simulink model "origin_cont"  (R2017b)
settings: Solver=VariableStepAuto  StartTime=0.0  StopTime=3  FixedStep=0.1  RelTol=1e-3
values from neighbouring files (symbols this model uses):
  gama1 = 109    [init.m]    (also in int.m = x(i,1); main.m = 10)
  gama2 = 2.04    [init.m]    (also in int.m = x(i,2); main.m = 10)
  kd = 3000    [PSO_main.m]    (also in init.m = 1000)
  ke = 1000    [PSO_main.m]    (also in init.m = 3000)
libraries: simulink x1
settings Model: Creator=Administrator  LastModifiedBy=Administrator
settings SolverCC: ZeroCrossAlgorithm=Adaptive
settings DebuggingCC: MaxConsecutiveZCsMsg=none
settings RTWCC: GenCodeOnly=on  PackageName=auto_impedance  Toolchain=Microsoft Visual C++ 2017 v15.0 | nmake (64-bit Windows)

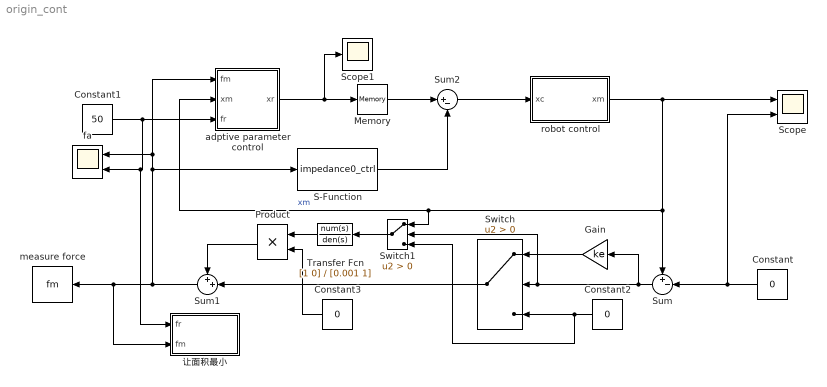
== system origin_cont ==
  Constant : Constant  Value=0
  Constant1 : Constant  Value=50
  Constant2 : Constant  Value=0
  Constant3 : Constant  Value=0
  Gain : Gain  Gain=ke
  Memory : Memory
  Product : Product
  S-Function : S-Function  FunctionName=impedance0_ctrl  Parameters=bd kd  SFunctionDeploymentMode=off  EnableBusSupport=off
  Scope : Scope  NumInputPorts=2
  Scope1 : Scope
  Sum : Sum  Inputs=+-|
  Sum1 : Sum  Inputs=++|
  Sum2 : Sum  Inputs=|+-
  Switch : Switch  Criteria=u2 > Threshold
  Switch1 : Switch  Criteria=u2 > Threshold
  Transfer Fcn : TransferFcn  Numerator=[1 0]  Denominator=[0.001 1]
  adptive parameter control : Subsystem
  fa : Scope  NumInputPorts=2
  "measure force " : ToWorkspace  VariableName=fm  SaveFormat=Timeseries  SampleTime=-1
  robot control : Subsystem
  让面积最小 : Subsystem
  wires:
  robot control/1("xm ") -> Switch1/1, adptive parameter control/2(xm), Sum/1, Scope/1  "xm"
  adptive parameter control/1(xr) -> Memory/1, Scope1/1
  Constant2/1 -> Switch1/3, Switch/3
  Sum2/1 -> robot control/1(xc)
  S-Function/1 -> Sum2/2
  Sum/1 -> Switch1/2, Switch/2, Gain/1
  Gain/1 -> Switch/1
  Constant1/1 -> 让面积最小/1(fr), fa/2, adptive parameter control/3(fr)
  Constant/1 -> Sum/2, Scope/2
  Sum1/1 -> fa/1, adptive parameter control/1(fm), S-Function/1, 让面积最小/2(fm), "measure force "/1
  Product/1 -> Sum1/1
  Transfer Fcn/1 -> Product/1
  Switch1/1 -> Transfer Fcn/1
  Switch/1 -> Sum1/2
  Constant3/1 -> Product/2
  Memory/1 -> Sum2/1

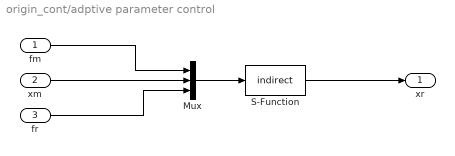
== system origin_cont/adptive parameter control ==
  fm : Inport
  xm : Inport  Port=2
  fr : Inport  Port=3
  Mux : Mux  Inputs=3
  S-Function : S-Function  FunctionName=indirect  Parameters=gama1 gama2 kd  SFunctionDeploymentMode=off  EnableBusSupport=off
  xr : Outport
  wires:
  fm/1 -> Mux/1
  xm/1 -> Mux/2
  Mux/1 -> S-Function/1
  fr/1 -> Mux/3
  S-Function/1 -> xr/1

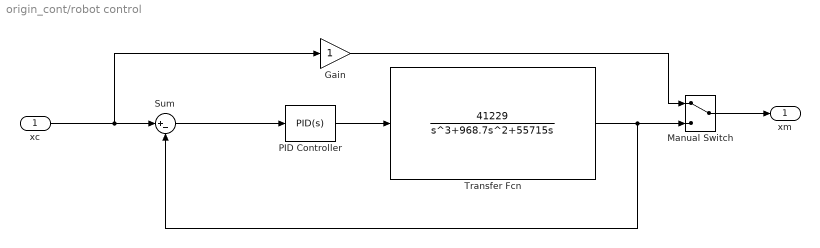
== system origin_cont/robot control ==
  xc : Inport
  Gain : Gain
  Manual Switch : ManualSwitch
  PID Controller : simulink/Continuous/PID Controller  Controller=PID  TimeDomain=Continuous-time  SampleTime=-1  IntegratorMethod=Forward Euler  FilterMethod=Forward Euler  Form=Parallel  UseFilter=on  ControllerParametersSource=internal  P=0.005  I=0.05  D=0.8  N=1  InitialConditionSource=internal  InitialConditionForIntegrator=0  InitialConditionForFilter=0  ExternalReset=none  LimitOutput=off  UpperSaturationLimit=inf  LowerSaturationLimit=-inf  LinearizeAsGain=on  AntiWindupMode=none  Kb=1  TrackingMode=off  Kt=1  PParamMin=[]  PParamMax=[]  IParamMin=[]  IParamMax=[]  DParamMin=[]  DParamMax=[]  NParamMin=[]  NParamMax=[]  KbParamMin=[]  KbParamMax=[]  KtParamMin=[]  KtParamMax=[]  POutMin=[]  POutMax=[]  IOutMin=[]  IOutMax=[]  DOutMin=[]  DOutMax=[]  NOutMin=[]  NOutMax=[]  KbOutMin=[]  KbOutMax=[]  KtOutMin=[]  KtOutMax=[]  IntegratorOutMin=[]  IntegratorOutMax=[]  FilterOutMin=[]  FilterOutMax=[]  SumOutMin=[]  SumOutMax=[]  SumI1OutMin=[]  SumI1OutMax=[]  SumI2OutMin=[]  SumI2OutMax=[]  SumI3OutMin=[]  SumI3OutMax=[]  SumDOutMin=[]  SumDOutMax=[]  SaturationOutMin=[]  SaturationOutMax=[]  IntegratorContinuousStateAttributes=''  IntegratorStateMustResolveToSignalObject=off  IntegratorRTWStateStorageClass=Auto  FilterContinuousStateAttributes=''  FilterStateMustResolveToSignalObject=off  FilterRTWStateStorageClass=Auto  DifferentiatorICPrevScaledInput=0  DifferentiatorOutMin=[]  DifferentiatorOutMax=[]  InitialConditionSetting=State (most efficient)  FilterDiffOutCoefMin=[]  FilterDiffOutCoefMax=[]  SumDenOutMin=[]  SumDenOutMax=[]  SumNumOutMin=[]  SumNumOutMax=[]  ReciprocalOutMin=[]  ReciprocalOutMax=[]  DivideOutMin=[]  DivideOutMax=[]  TunerSelectOption=Transfer Function Based (PID Tuner App)
  Sum : Sum  Inputs=|+-
  Transfer Fcn : TransferFcn  Numerator=[41229]  Denominator=[1 968.7 55715 0]
  "xm " : Outport
  wires:
  Sum/1 -> PID Controller/1
  xc/1 -> Gain/1, Sum/1
  Manual Switch/1 -> "xm "/1
  PID Controller/1 -> Transfer Fcn/1
  Transfer Fcn/1 -> Sum/2, Manual Switch/2
  Gain/1 -> Manual Switch/1

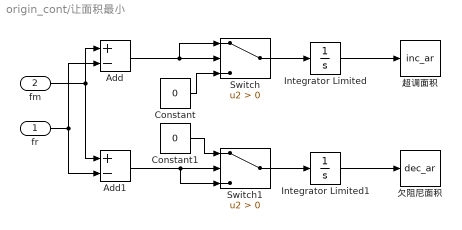
== system origin_cont/让面积最小 ==
  fr : Inport
  fm : Inport  Port=2
  " 欠阻尼面积" : ToWorkspace  VariableName=dec_ar  SaveFormat=Timeseries  SampleTime=-1
  Add : Sum  Inputs=+-
  Add1 : Sum  Inputs=+-
  Constant : Constant  Value=0
  Constant1 : Constant  Value=0
  Integrator Limited : Integrator  UpperSaturationLimit=1  LowerSaturationLimit=0  ZeroCross=off
  Integrator Limited1 : Integrator  UpperSaturationLimit=1  LowerSaturationLimit=0  ZeroCross=off
  Switch : Switch  Criteria=u2 > Threshold
  Switch1 : Switch  Criteria=u2 > Threshold
  "超调面积 " : ToWorkspace  VariableName=inc_ar  SaveFormat=Timeseries  SampleTime=-1
  wires:
  Switch/1 -> Integrator Limited/1
  fm/1 -> Add/1, Add1/1
  fr/1 -> Add/2, Add1/2
  Add/1 -> Switch/1, Switch/2
  Constant/1 -> Switch/3
  Add1/1 -> Switch1/3, Switch1/2
  Switch1/1 -> Integrator Limited1/1
  Constant1/1 -> Switch1/1
  Integrator Limited/1 -> "超调面积 "/1
  Integrator Limited1/1 -> " 欠阻尼面积"/1
